simulink model "te_test"  (Simulink 5.0)
settings: Solver=ode45  SolverMode=SingleTasking  StartTime=0.0  StopTime=3  FixedStep=1/3600  MaxStep=1/60  RelTol=1e-3
StopFcn:
  | teplot
settings Model: LastModifiedBy=Administrator  SaveOutput=off  LimitDataPoints=off  BooleanDataType=off

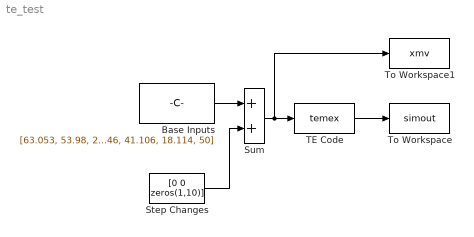
== system te_test ==
  Base Inputs : Constant  Value=[63.053, 53.98, 24.644, 61.302, 22.21, 40.064, 38.10, 46.534, 47.446, 41.106, 18.114, 50]
  Step Changes : Constant  Value="[0 0  zeros(1,10)]"
  Sum : Sum  SaturateOnIntegerOverflow=on  InputSameDT=on
  TE Code : S-Function  FunctionName=temex  Parameters=[], [zeros(1,7), 0, zeros(1,12)]
  To Workspace : ToWorkspace  VariableName=simout  SampleTime=-1  SaveFormat=Array
  To Workspace1 : ToWorkspace  VariableName=xmv  SampleTime=-1  SaveFormat=Array
  wires:
  TE Code/1 -> To Workspace/1
  Base Inputs/1 -> Sum/1
  Sum/1 -> TE Code/1, To Workspace1/1
  Step Changes/1 -> Sum/2
